simulink library "INT_Diff_TrqRat"  (R2016b)
settings: Solver=VariableStepAuto  StartTime=0.0  StopTime=10.0  RelTol=1e-3
settings Model: Creator=Administrator  LastModifiedBy=Administrator

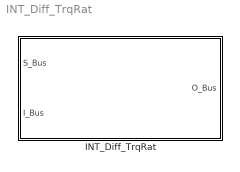
== system INT_Diff_TrqRat ==
  INT_Diff_TrqRat : Subsystem

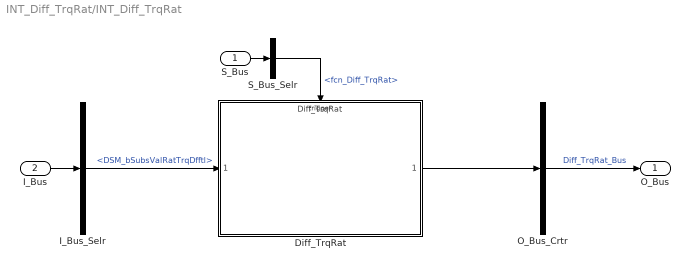
== system INT_Diff_TrqRat/INT_Diff_TrqRat ==
  S_Bus : Inport
  I_Bus : Inport  Port=2
  Diff_TrqRat : ModelReference  ModelNameDialog=Diff_TrqRat  SimulationMode=Normal  ModelReferenceVersion=1.5  TriggerPortName=function  TriggerPortTriggerType=function-call  TriggerPortStatesWhenEnabling=held
  I_Bus_Selr : BusSelector  OutputSignals=DSM_bSubsValRatTrqDfftl
  O_Bus_Crtr : BusCreator  Inputs=1
  S_Bus_Selr : BusSelector  OutputSignals=fcn_Diff_TrqRat
  O_Bus : Outport
  wires:
  S_Bus_Selr/1 -> Diff_TrqRat/Trigger  "<fcn_Diff_TrqRat>"
  S_Bus/1 -> S_Bus_Selr/1
  I_Bus/1 -> I_Bus_Selr/1
  I_Bus_Selr/1 -> Diff_TrqRat/1  "<DSM_bSubsValRatTrqDfftl>"
  O_Bus_Crtr/1 -> O_Bus/1  "Diff_TrqRat_Bus"
  Diff_TrqRat/1 -> O_Bus_Crtr/1
